simulink model "SimpleBatteryModel_Sim"  (R2022b)
settings: Solver=VariableStepAuto  StartTime=0.0  StopTime=Sim_time  RelTol=1e-3
values from neighbouring files (symbols this model uses):
  I = 2.3    [SimpleBatteryModeling.m]
  Q = 2.3*3600    (= 8280)    [SimpleBatteryModeling.m]
  R_charge = Data(:,3)    [SimpleBatteryModeling.m]
  R_discharge = Data(:,4)    [SimpleBatteryModeling.m]
  SoC = Data(:,1)    [SimpleBatteryModeling.m]
settings Model: Creator=koush  LastModifiedBy=koush

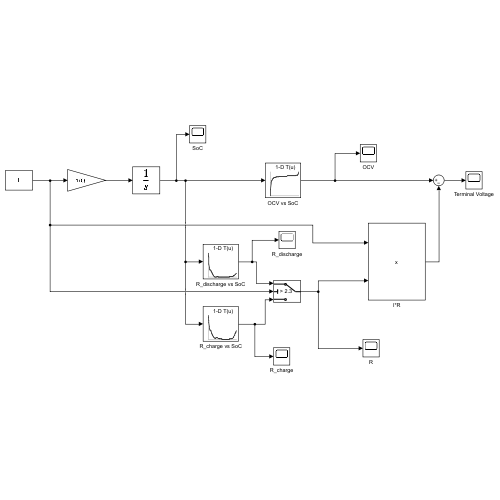
[thumbnail: Simulink's stored preview of the top-level diagram]
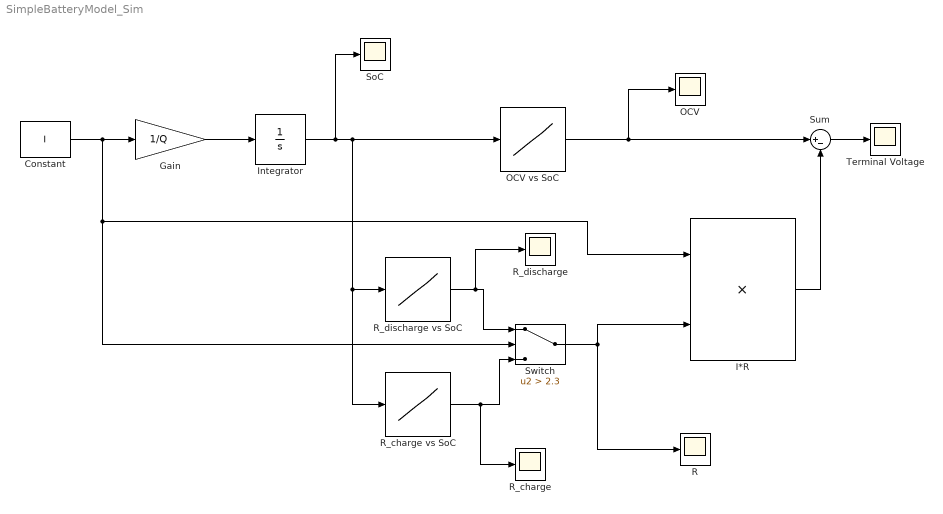
== system SimpleBatteryModel_Sim ==
  Constant : Constant  Value=I
  Gain : Gain  Gain=1/Q
  I*R : Product
  Integrator : Integrator
  OCV : Scope
  OCV vs SoC : Lookup_n-D  NumberOfTableDimensions=1  BreakpointsForDimension1=[0;0.01;0.02;0.03;0.04;0.05;0.06;0.07;0.08;0.09;0.1;0.11;0.12;0.13;0.14;0.15;0.16;0.17;0.18;0.19;0.2;0.21;0.22;0.23;0.24;0.25;0.26;0.27;0.28;0.29;0.3;0.31;0.32;0.33;0.34;0.35;0.36;0.37;0.38;0.39;0.4;0.41;0.42;0.43;0.44;0.45;0.46;0.47;0.48;0.49;0.5;0.51;0.52;0.53;0.54;0.55;0.56;0.57;0.58;0.59;0.6;0.61;0.62;0.63;0.64;0.65;0.66;0.67;0.68;0.69;0.7;0.71;0.72;0.73;0.74;0.75;0.76;0.77;0.78;0.79;0.8;0.81;0.82;0.83;0.84;0.85;0.86;0.87;0.88;0.89;0.9;0.91;0.92;0.93;0.94;0.95;0.96;0.97;0.98;0.99;1]  Table=[2.4;2.86404;3.33456;3.47124;3.5586;3.62364;3.6762;3.72036;3.7584;3.7902;3.81708;3.83568;3.84504;3.8508;3.85596;3.861;3.867;3.87528;3.88308;3.88956;3.89496;3.89976;3.9048;3.90828;3.9132;3.91788;3.92184;3.92652;3.92964;3.93192;3.93552;3.93828;3.94092;3.94296;3.94644;3.9486;3.9498;3.95256;3.95436;3.95616;3.95796;3.95904;3.9588;3.96048;3.96144;3.9624;3.96324;3.96372;3.9648;3.96588;3.96636;3.96792;3.969;3.97092;3.97296;3.97356;3.97512;3.97704;3.97872;3.97944;3.98112;3.9858;3.98724;3.98964;3.99192;3.99432;3.99636;3.99876;4.00032;4.00224;4.00452;4.00572;4.0068;4.008;4.00884;4.00992;4.01028;4.01052;4.01088;4.0116;4.01244;4.01245;4.01364;4.01448;4.01508;4.0158;4.01628;4.01784;4.01928;4.02108;4.02264;4.02516;4.02708;4.03128;4.03584;4.04376;4.05624;4.07772;4.11816;4.19436;4.32]  InternalRulePriority=Speed  RndMeth=Simplest
  R : Scope
  R_charge : Scope
  R_charge vs SoC : Lookup_n-D  NumberOfTableDimensions=1  BreakpointsForDimension1=SoC  Table=R_charge  InternalRulePriority=Speed  RndMeth=Simplest
  R_discharge : Scope
  R_discharge vs SoC : Lookup_n-D  NumberOfTableDimensions=1  BreakpointsForDimension1=SoC  Table=R_discharge  InternalRulePriority=Speed  RndMeth=Simplest
  SoC : Scope
  Sum : Sum  Inputs=|+-
  Switch : Switch  Criteria=u2 > Threshold  Threshold=2.3  SaturateOnIntegerOverflow=off  InputSameDT=off
  Terminal Voltage : Scope
  wires:
  Gain/1 -> Integrator/1
  Constant/1 -> Switch/2, I*R/1, Gain/1
  Integrator/1 -> OCV vs SoC/1, R_charge vs SoC/1, R_discharge vs SoC/1, SoC/1
  OCV vs SoC/1 -> OCV/1, Sum/1
  Sum/1 -> Terminal Voltage/1
  I*R/1 -> Sum/2
  R_discharge vs SoC/1 -> R_discharge/1, Switch/1
  R_charge vs SoC/1 -> R_charge/1, Switch/3
  Switch/1 -> R/1, I*R/2
